simulink subsystem "False_Data_Injection_Model"  (R2023b)
settings: Solver=VariableStepAuto  StartTime=0.0  StopTime=10.0  RelTol=1e-3
settings Model: Creator=20155555  LastModifiedBy=20155555

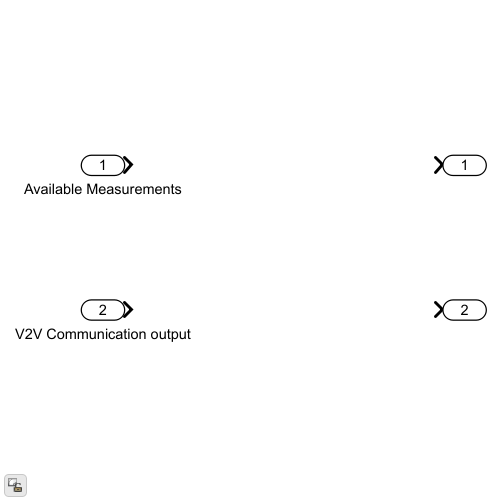
[thumbnail: Simulink's stored preview of the top-level diagram]
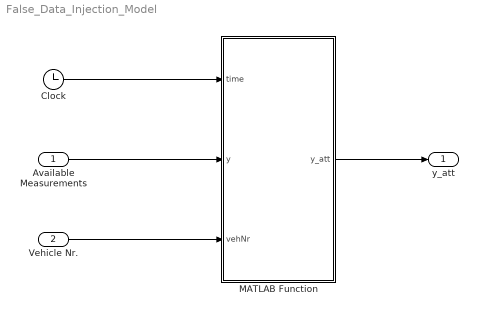
== system False_Data_Injection_Model ==
  Available Measurements : Inport
  Vehicle Nr. : Inport  Port=2
  Clock : Clock
  MATLAB Function : MATLAB Function  TreatAsAtomicUnit=on
  y_att : Outport
  wires:
  Vehicle Nr./1 -> MATLAB Function/3(vehNr)
  Available Measurements/1 -> MATLAB Function/2(y)
  Clock/1 -> MATLAB Function/1(time)
  MATLAB Function/1(y_att) -> y_att/1

== matlab function False_Data_Injection_Model/MATLAB Function ==
  data: time input; y input; y_att output; vehNr input; simulation parameter
function y_att = fcn(time, y, vehNr, simulation)

y1 = y(1);
y2 = y(2);
% y3 = y(3);
% y4 = y(4);
y5a = y(5);
y5b = y(5);
y6a = y(6);
y6b = y(6);

if vehNr == simulation.attack.vehAtt

    if simulation.att_5a_start1 <= time && time < simulation.att_5a_end1
        y_att = [y1; y2; y5a + cos(25*time); 
            y5b; y6a; y6b];

    elseif simulation.att_5a_start2 <= time && time < simulation.att_5a_end2
        y_att = [y1; y2; y5a + exp(0.1*time)+sin(10*time); 
            y5b; y6a; y6b];

    elseif simulation.att_5b_start <= time && time < simulation.att_5b_end
        y_att = [y1; y2; y5a; y5b + cos(time); 
            y6a; y6b];

    elseif simulation.att_6a_start <= time && time < simulation.att_6a_end
        y_att = [y1; y2; y5a; y5b; y6a + exp(0.3*time); 
            y6b];

    elseif simulation.att_6b_start <= time && time < simulation.att_6b_end
        y_att = [y1; y2; y5a; y5b; y6a; y6b + 2*cos(10*time)];

    else
        y_att = [y1; y2; y5a; y5b; y6a; y6b];
    end

else

    y_att = [y1; y2; y5a; y5b; y6a; y6b];

end
